simulink model "seventh"  (R2021b)
settings: Solver=ode23s  StartTime=0.0  StopTime=30  RelTol=1e-3
libraries: spsGroundLib x4, spsCurrentMeasurementLib x3, spsDCMachineLib x2, spsDCVoltageSourceLib x2, spsIdealSwitchLib x2, spsSeriesRLCBranchLib x2, spsVoltageMeasurementLib x2, spspowerguiLib x1
settings Model: Creator=minna  LastModifiedBy=minna
settings SolverCC: ZeroCrossAlgorithm=Adaptive
settings DebuggingCC: IgnoredZcDiagnostic=none

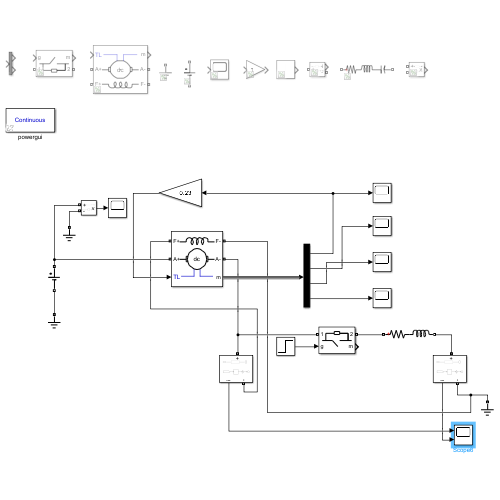
[thumbnail: Simulink's stored preview of the top-level diagram]
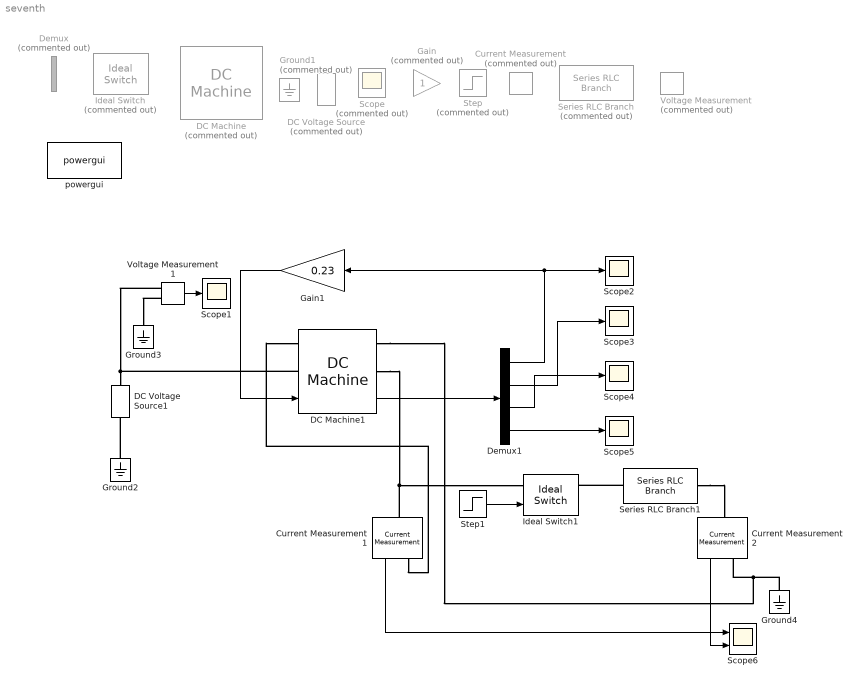
== system seventh ==
  Current Measurement : spsCurrentMeasurementLib/Current Measurement  Commented=on  PhasorSimulation=off  OutputType=Complex  PSBequivalent=0
  Current Measurement1 : spsCurrentMeasurementLib/Current Measurement  PhasorSimulation=off  OutputType=Complex  PSBequivalent=0
  Current Measurement2 : spsCurrentMeasurementLib/Current Measurement  PhasorSimulation=off  OutputType=Complex  PSBequivalent=0
  DC Machine : spsDCMachineLib/DC Machine  Commented=on  PresetModel=No  MechanicalLoad=Torque TL  FieldType=Wound  ShowDetailedParameters=on  MeasurementBus=off  RLa="[ 0.6  0.012]"  RLf="[ 240  120]"  Laf=1.8  MachineConstant=Torque constant (N.m/A)  Ke=1.8  Kt=1.8  J=1  Bm=0  Tf=0  w0=1  Ifinit=1  TsPowergui=0  TsBlock=-1
  DC Machine1 : spsDCMachineLib/DC Machine  PresetModel=No  MechanicalLoad=Torque TL  FieldType=Wound  ShowDetailedParameters=on  MeasurementBus=off  RLa="[ 0.6717  0.001882]"  RLf="[ 30.72  3.166]"  Laf=0.2641  MachineConstant=Torque constant (N.m/A)  Ke=1.8  Kt=1.8  J=1.019  Bm=0  Tf=26.46  w0=1  Ifinit=7.48600604818369  TsPowergui=0  TsBlock=-1
  DC Voltage Source : spsDCVoltageSourceLib/DC Voltage Source  Commented=on  Amplitude=100  Measurements=None
  DC Voltage Source1 : spsDCVoltageSourceLib/DC Voltage Source  Amplitude=235  Measurements=None
  Demux : Demux  Commented=on  Outputs=2
  Demux1 : Demux
  Gain : Gain  Commented=on
  Gain1 : Gain  Gain=0.23
  Ground1 : spsGroundLib/Ground  Commented=on  LConnTagsString=a
  Ground2 : spsGroundLib/Ground  LConnTagsString=a
  Ground3 : spsGroundLib/Ground  LConnTagsString=a
  Ground4 : spsGroundLib/Ground  LConnTagsString=a
  Ideal Switch : spsIdealSwitchLib/Ideal Switch  Commented=on  Ron=0.001  Lon=0  IC=0  Rs=1e5  Cs=inf  Measurements=on
  Ideal Switch1 : spsIdealSwitchLib/Ideal Switch  Ron=0.0001  Lon=0  IC=0  Rs=1e5  Cs=inf  Measurements=on
  Scope : Scope  Commented=on
  Scope{1..5} (5 alike) : Scope
  Scope6 : Scope  NumInputPorts=2
  Series RLC Branch : spsSeriesRLCBranchLib/Series RLC Branch  Commented=on  LConnTagsString=__new0  RConnTagsString=__new0  BranchType=RLC  Resistance=1  Inductance=1e-3  SetiL0=off  InitialCurrent=0  Capacitance=1e-6  Setx0=off  InitialVoltage=0  Measurements=None
  Series RLC Branch1 : spsSeriesRLCBranchLib/Series RLC Branch  LConnTagsString=__new0  RConnTagsString=__new0  BranchType=RL  Resistance=50  Inductance=15.5  SetiL0=off  InitialCurrent=0  Capacitance=1e-6  Setx0=off  InitialVoltage=0  Measurements=None
  Step : Step  Commented=on  SampleTime=0
  Step1 : Step  Time=10  SampleTime=0
  Voltage Measurement : spsVoltageMeasurementLib/Voltage Measurement  Commented=on  PhasorSimulation=off  OutputType=Complex  PSBequivalent=0
  Voltage Measurement1 : spsVoltageMeasurementLib/Voltage Measurement  PhasorSimulation=off  OutputType=Complex  PSBequivalent=0
  powergui : spspowerguiLib/powergui  Priority=1  SimulationMode=Continuous  SampleTime=50e-6  frequency=60  Iterations=50  frequencyindice=0  Pbase=100e6  ErrMax=1e-4  UnitsV=kV  UnitsW=MW  buscounter=0  FunctionMessages=off  echomessages=off  EnableUseOfTLC=off  CurrentSourceSwitches=off  DisableSnubberDevices=off  DisableRonSwitches=off  DisableVfSwitches=off  DisplayEquations=off  AutomaticDiscreteSolvers=off  SolverType=Tustin/Backward Euler (TBE)  Interpol=off  ExternalGateDelay=off  methode=off  Ts=100  x0status=blocks  SPID=on  SwTol=0  HookPort=off  NonlinearTolerance=1e-4  nMaxIteration=100  ContinueOnMaxIteration=off  RestoreLinks=warning  ResistiveCurrentMeasurement=off  Frange=[0:2:500]  Ylog=off  Xlog=on  ShowGrid=off  save=off  variable=ZData  structure=0  ZoomFFT=off  StartTime=0.0  cycles=1  DisplayStyle=1  fundamental=60  FreqAxis=off  MaxFrequency=1000  frequencyindicesteady=1  RmsSteady=1  display=off
  wires:
  Voltage Measurement1/1 -> Scope1/1
  DC Machine1/1 -> Demux1/1
  Demux1/1 -> Gain1/1, Scope2/1
  Demux1/2 -> Scope3/1
  Demux1/3 -> Scope4/1
  Demux1/4 -> Scope5/1
  Gain1/1 -> DC Machine1/1
  Step1/1 -> Ideal Switch1/1
  Current Measurement2/1 -> Scope6/2
  Current Measurement1/1 -> Scope6/1
  connections:
  Ground2/LConn1 -- DC Voltage Source1/LConn1
  Voltage Measurement1/LConn2 -- Ground3/LConn1
  Voltage Measurement1/LConn1 -- DC Machine1/LConn1 -- DC Voltage Source1/RConn1
  DC Machine1/RConn1 -- Current Measurement1/LConn1 -- Ideal Switch1/LConn1
  Series RLC Branch1/LConn1 -- Ideal Switch1/RConn1
  Current Measurement1/RConn1 -- DC Machine1/LConn2
  Series RLC Branch1/RConn1 -- Current Measurement2/LConn1
  Ground4/LConn1 -- DC Machine1/RConn2 -- Current Measurement2/RConn1
